simulink model "db2"  (R2018a)
settings: Solver=VariableStepAuto  StartTime=0.0  StopTime=10.0  MaxStep=1e-3  RelTol=1e-3
values from neighbouring files (symbols this model uses):
  bg = 4    [codigo.m]
  bm = 1    [codigo.m]
  Jm = 1    [codigo.m]
  kb = 1    [codigo.m]
  ki = 1    [codigo.m]
  M = 1    [codigo.m]
  n1 = 1    [codigo.m]
  n2 = 10    [codigo.m]
  R = 2    [codigo.m]
  Ra = 1    [codigo.m]
settings Model: Creator=carma  LastModifiedBy=carma

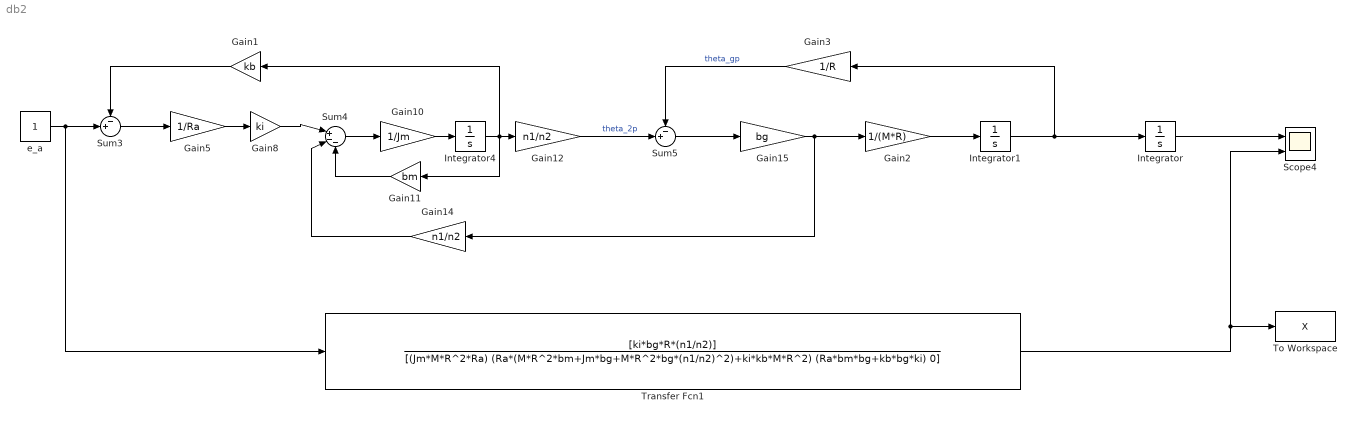
== system db2 ==
  Gain1 : Gain  Gain=kb
  Gain10 : Gain  Gain=1/Jm
  Gain11 : Gain  Gain=bm
  Gain12 : Gain  Gain=n1/n2
  Gain14 : Gain  Gain=n1/n2
  Gain15 : Gain  Gain=bg
  Gain2 : Gain  Gain=1/(M*R)
  Gain3 : Gain  Gain=1/R
  Gain5 : Gain  Gain=1/Ra
  Gain8 : Gain  Gain=ki
  Integrator : Integrator
  Integrator1 : Integrator
  Integrator4 : Integrator
  Scope4 : Scope  NumInputPorts=2
  Sum3 : Sum  Inputs=-+|
  Sum4 : Sum  Inputs=|+--
  Sum5 : Sum  Inputs=-+|
  To Workspace : ToWorkspace  VariableName=X  SampleTime=1e-3
  Transfer Fcn1 : TransferFcn  Numerator=[ki*bg*R*(n1/n2)]  Denominator=[(Jm*M*R^2*Ra) (Ra*(M*R^2*bm+Jm*bg+M*R^2*bg*(n1/n2)^2)+ki*kb*M*R^2) (Ra*bm*bg+kb*bg*ki) 0]
  e_a : Constant
  wires:
  Integrator1/1 -> Gain3/1, Integrator/1
  Gain5/1 -> Gain8/1
  Sum3/1 -> Gain5/1
  Gain10/1 -> Integrator4/1
  Gain11/1 -> Sum4/3
  Gain8/1 -> Sum4/1
  Sum5/1 -> Gain15/1
  Integrator4/1 -> Gain1/1, Gain11/1, Gain12/1
  Gain14/1 -> Sum4/2
  Sum4/1 -> Gain10/1
  e_a/1 -> Transfer Fcn1/1, Sum3/2
  Gain1/1 -> Sum3/1
  Gain15/1 -> Gain14/1, Gain2/1
  Gain2/1 -> Integrator1/1
  Gain12/1 -> Sum5/2  "theta_2p"
  Gain3/1 -> Sum5/1  "theta_gp"
  Integrator/1 -> Scope4/1
  Transfer Fcn1/1 -> To Workspace/1, Scope4/2
